simulink model "A13_Servoachse_Nyquist"  (R2017b)
settings: Solver=ode45  StartTime=0.0  StopTime=20  FixedStep=0.001  MaxStep=1E-3  RelTol=1e-3  EnableMultiTasking=on
values from neighbouring files (symbols this model uses):
  CF = 1e4    (= 10000)    [A13_Konstanten.m]    (also in A14_Konstanten.m; A17_Konstanten.m = 50000; A8_Konstanten.m = 10000000; A9_Konstanten.m)
  CM = 7.1e-7    (= 7.1e-07)    [A10_Konstanten.m]    (also in A13_Konstanten.m; A14_Konstanten.m; A16_Konstanten.m)
  CR = 0.2    [A13_Konstanten.m]    (also in A14_Konstanten.m; A17_Konstanten.m = 100; A9_Konstanten.m = 1; Z_Parametrisierung_Skript.m = [0.5,1,5])
  FReib = 0.5    [A13_Konstanten.m]    (also in A14_Konstanten.m)
  JM = JR + JG    (= 1.38e-06)    [A13_Konstanten.m]    (also in A14_Konstanten.m)
  JR = 1.32e-6    (= 1.32e-06)    [A10_Konstanten.m]    (also in A13_Konstanten.m; A14_Konstanten.m; A16_Konstanten.m; A9_Konstanten.m = 0.004)
  KM = 38.4e-3    (= 0.0384)    [A10_Konstanten.m]    (also in A13_Konstanten.m; A14_Konstanten.m; A16_Konstanten.m)
  KN = 1/(2*pi*KM)    (= 4.14465997635)    [A10_Konstanten.m]    (also in A13_Konstanten.m; A14_Konstanten.m; A16_Konstanten.m)
  LA = 4.64e-4    (= 0.000464)    [A10_Konstanten.m]    (also in A13_Konstanten.m; A14_Konstanten.m; A16_Konstanten.m)
  m1 = 1    [A13_Konstanten.m]    (also in A14_Konstanten.m; A17_Konstanten.m = 4; A8_Konstanten.m = 20)
  R = 0.02    [A10_Konstanten.m]    (also in A13_Konstanten.m = 0.04; A14_Konstanten.m = 0.04; A16_Konstanten.m)
  RA = 4.99    [A10_Konstanten.m]    (also in A13_Konstanten.m; A14_Konstanten.m; A16_Konstanten.m)
  Ue = 4    [A13_Konstanten.m]    (also in A14_Konstanten.m)
  UN = 24    [A13_Konstanten.m]    (also in A14_Konstanten.m)
  WGrad = 0.85    [A13_Konstanten.m]    (also in A14_Konstanten.m)
undefined symbols (not defined in the file or in its folder): sigbuilder_block
libraries: simulink x1
settings Model: Creator=jbaur  LastModifiedBy=lukasschwoerer
settings DataIOCC: ExternalInput=X1  SaveFormat=StructureWithTime  InspectSignalLogs=on  SignalLoggingName=sigsOut
settings OptimizationCC: DefaultParameterBehavior=Inlined  InlineInvariantSignals=on  BufferReuse=off  ExpressionDepthLimit=2147483647  InitFltsAndDblsToZero=on  LifeSpan=inf
settings DebuggingCC: SaveWithParameterizedLinksMsg=none  SignalResolutionControl=TryResolveAllWithWarning  MultiTaskDSMMsg=warning  MultiTaskCondExecSysMsg=none  StateNameClashWarn=warning  InitInArrayFormatMsg=none  SFUnexpectedBacktrackingDiag=warning  SFNoUnconditionalDefaultTransitionDiag=warning  SFExecutionAtInitializationDiag=none
settings HardwareCC: ProdBitPerPointer=32  ProdBitPerSizeT=32  ProdBitPerPtrDiffT=32  ProdLargestAtomicFloat=None  ProdIntDivRoundTo=Undefined  ProdEndianess=Unspecified  ProdWordSize=32  ProdHWDeviceType=32-bit Generic  TargetUnknown=on
settings ModelReferenceCC: PropagateSignalLabelsOutOfModel=off
settings CodeAppCC: StateflowObjectComments=on
settings GRTTargetCC: TargetFcnLib=ansi_tfl_tmw.mat  TargetLangStandard=C89/C90 (ANSI)  ModelReferenceCompliant=off  GeneratePreprocessorConditionals=Disable all  CombineOutputUpdateFcns=off  MatFileLogging=off  GRTInterface=on
settings ConfigComp: CovMetricSettings=dw  CovHtmlReporting=on  CovSaveCumulativeToWorkspaceVar=on  CovSaveSingleToWorkspaceVar=on  CovExternalEMLEnable=off  CovSFcnEnable=off

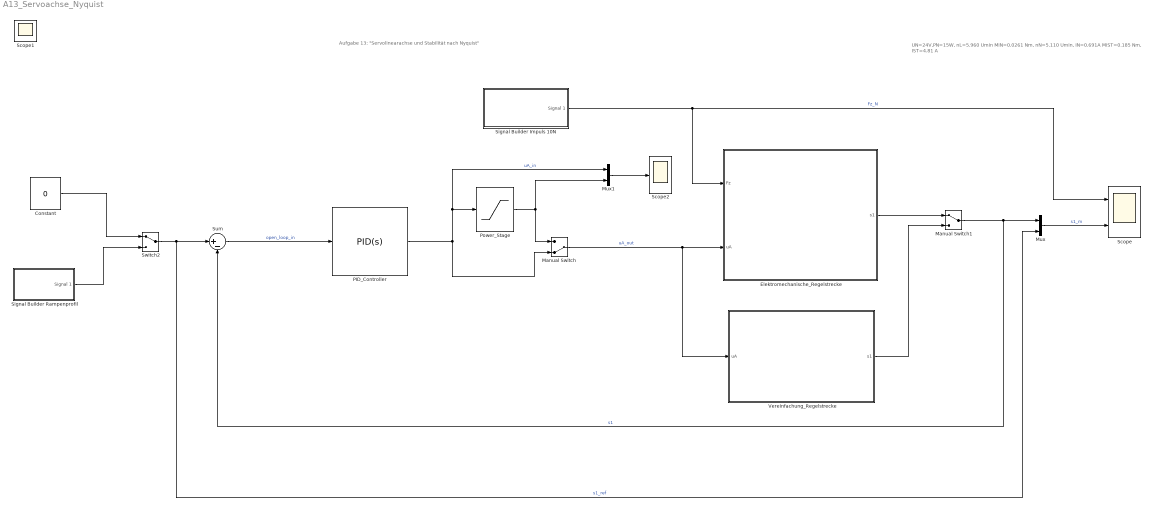
== system A13_Servoachse_Nyquist ==
  note: Aufgabe 13: "Servolinearachse und Stabilität nach Nyquist"
  note: UN=24V,PN=15W, nL=5.960 Umin
      | MiN=0.0261 Nm, nN=5.110 Umin, IN=0.691A
      | MiST=0.185 Nm, IST=4.81 A
  Constant : Constant  Value=0
  Elektromechanische_Regelstrecke : Subsystem
  Manual Switch : ManualSwitch  CurrentSetting=0
  Manual Switch1 : ManualSwitch
  Mux : Mux  Inputs=2
  Mux1 : Mux  Inputs=2
  PID_Controller : simulink/Continuous/PID Controller  Controller=PID  TimeDomain=Continuous-time  SampleTime=-1  IntegratorMethod=Forward Euler  FilterMethod=Forward Euler  Form=Ideal  UseFilter=on  ControllerParametersSource=internal  P=2480.03319241958  I=4.7969020161188  D=0.0477426789872327  N=295.112462731563  InitialConditionSource=internal  InitialConditionForIntegrator=0  InitialConditionForFilter=0  ExternalReset=none  LimitOutput=off  UpperSaturationLimit=UN  LowerSaturationLimit=-UN  LinearizeAsGain=off  AntiWindupMode=none  Kb=1  TrackingMode=off  Kt=1  PParamMin=[]  PParamMax=[]  IParamMin=[]  IParamMax=[]  DParamMin=[]  DParamMax=[]  NParamMin=[]  NParamMax=[]  KbParamMin=[]  KbParamMax=[]  KtParamMin=[]  KtParamMax=[]  POutMin=[]  POutMax=[]  IOutMin=[]  IOutMax=[]  DOutMin=[]  DOutMax=[]  NOutMin=[]  NOutMax=[]  KbOutMin=[]  KbOutMax=[]  KtOutMin=[]  KtOutMax=[]  IntegratorOutMin=[]  IntegratorOutMax=[]  FilterOutMin=[]  FilterOutMax=[]  SumOutMin=[]  SumOutMax=[]  SumI1OutMin=[]  SumI1OutMax=[]  SumI2OutMin=[]  SumI2OutMax=[]  SumI3OutMin=[]  SumI3OutMax=[]  SumDOutMin=[]  SumDOutMax=[]  SaturationOutMin=[]  SaturationOutMax=[]  IntegratorContinuousStateAttributes=''  IntegratorStateMustResolveToSignalObject=off  IntegratorRTWStateStorageClass=Auto  FilterContinuousStateAttributes=''  FilterStateMustResolveToSignalObject=off  FilterRTWStateStorageClass=Auto  DifferentiatorICPrevScaledInput=0  DifferentiatorOutMin=[]  DifferentiatorOutMax=[]  InitialConditionSetting=State (most efficient)  FilterDiffOutCoefMin=[]  FilterDiffOutCoefMax=[]  SumDenOutMin=[]  SumDenOutMax=[]  SumNumOutMin=[]  SumNumOutMax=[]  ReciprocalOutMin=[]  ReciprocalOutMax=[]  DivideOutMin=[]  DivideOutMax=[]  TunerSelectOption=Transfer Function Based (PID Tuner App)
  Power_Stage : Saturate  UpperLimit=UN  LowerLimit=-UN
  Scope : Scope  NumInputPorts=2
  Scope2 : Scope
  Signal Builder Impuls 10N : Subsystem  Tag=STV Subsys  LoadFcn=sigbuilder_block('load');  StartFcn=sigbuilder_block('start');  StopFcn=sigbuilder_block('stop');  ClipboardFcn=sigbuilder_block('clipboard');  mask(Sigbuilder block){tuvar=[0:10]}
      mask help: Simulink:masks:SigbuilderBlock_MD
      mask init:
      | if ~strcmp(get_param(bdroot(gcbh),'SimulationStatus'),'stopped') tuvar = sigbuilder_block('maskInit'); end
      settings: CopyFcn=sigbuilder_block('copy');  DeleteFcn=sigbuilder_block('delete');  ModelCloseFcn=sigbuilder_block('modelClose');  PreSaveFcn=sigbuilder_block('preSave');  PauseFcn=sigbuilder_block('pause');  ContinueFcn=sigbuilder_block('continue');  NameChangeFcn=sigbuilder_block('namechange');  OpenFcn=sigbuilder_block('open',[437 199 551 400 ]);  CloseFcn=sigbuilder_block('close');
      mask Display: plot(0, 0, 100, 100,[2, 2, 32, 32, 2], [68, 8, 8, 68, 68],[32, 2], [38, 38], [32, 19, 2],[53, 60, 44], [32, 17, 17, 2],[16, 16, 31, 31]);txt = getActiveGroup(gcbh);text(2, 100, txt,'verticalAlignment', 'top');
  Signal Builder Rampenprofil : Subsystem  Tag=STV Subsys  LoadFcn=sigbuilder_block('load');  StartFcn=sigbuilder_block('start');  StopFcn=sigbuilder_block('stop');  ClipboardFcn=sigbuilder_block('clipboard');  mask(Sigbuilder block){tuvar=[0:10]}
      mask help: Create and generate interchangeable groups of signals whose waveforms are piecewise linear.
      mask init:
      | if ~strcmp(get_param(bdroot(gcbh),'SimulationStatus'),'stopped') tuvar = sigbuilder_block('maskInit'); end
      settings: CopyFcn=sigbuilder_block('copy');  DeleteFcn=sigbuilder_block('delete');  ModelCloseFcn=sigbuilder_block('modelClose');  PreSaveFcn=sigbuilder_block('preSave');  PauseFcn=sigbuilder_block('pause')  ContinueFcn=sigbuilder_block('continue')  NameChangeFcn=sigbuilder_block('namechange');  OpenFcn=sigbuilder_block('open',[441.75 165.75 550.5 399.75 ]);  CloseFcn=sigbuilder_block('close');
      mask Display: plot(0, 0, 100, 100,[2, 2, 32, 32, 2], [68, 8, 8, 68, 68],[32, 2], [38, 38], [32, 19, 2],[53, 60, 44], [32, 17, 17, 2],[16, 16, 31, 31]);txt = getActiveGroup(gcbh);text(2, 100, txt,'verticalAlignment', 'top');
  Sum : Sum  Inputs=|+-  SaturateOnIntegerOverflow=on
  Switch2 : ManualSwitch
  Vereinfachung_Regelstrecke : Subsystem
  Scope1 : Scope
  wires:
  Sum/1 -> PID_Controller/1  "open_loop_in"
  Signal Builder Impuls 10N/1(Signal 1) -> Elektromechanische_Regelstrecke/1(Fz), Scope/1  "Fz_N"
  Switch2/1 -> Sum/1, Mux/2  "s1_ref"
  Constant/1 -> Switch2/1
  Signal Builder Rampenprofil/1(Signal 1) -> Switch2/2
  Mux/1 -> Scope/2  "s1_m"
  Power_Stage/1 -> Manual Switch/1, Mux1/2
  Manual Switch/1 -> Vereinfachung_Regelstrecke/1(uA), Elektromechanische_Regelstrecke/2(uA)  "uA_out"
  PID_Controller/1 -> Manual Switch/2, Mux1/1, Power_Stage/1  "uA_in"
  Mux1/1 -> Scope2/1
  Manual Switch1/1 -> Sum/2, Mux/1  "s1"
  Elektromechanische_Regelstrecke/1(s1) -> Manual Switch1/1
  Vereinfachung_Regelstrecke/1(s1) -> Manual Switch1/2

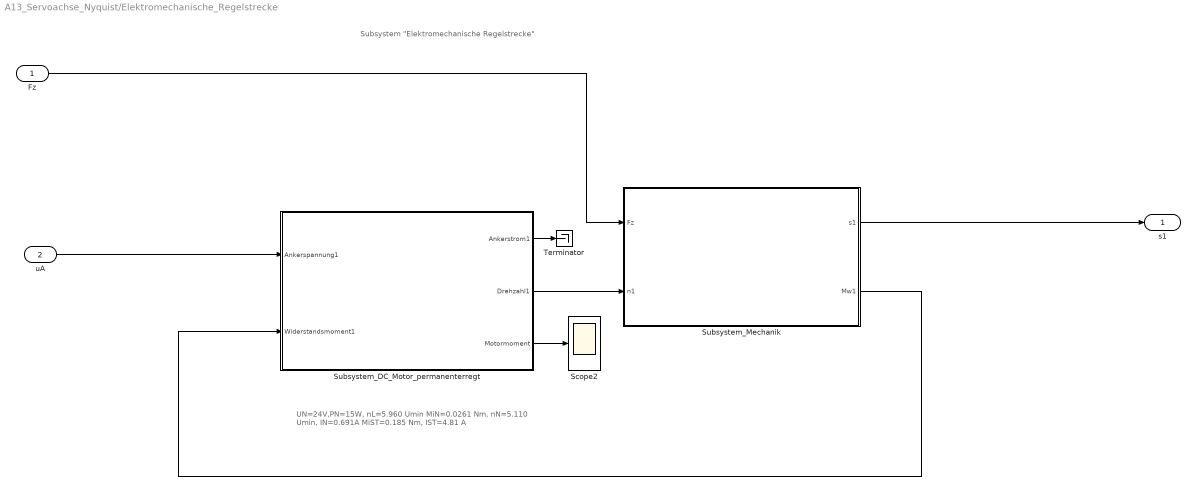
== system A13_Servoachse_Nyquist/Elektromechanische_Regelstrecke ==
  note: Subsystem "Elektromechanische Regelstrecke"
  note: UN=24V,PN=15W, nL=5.960 Umin
      | MiN=0.0261 Nm, nN=5.110 Umin, IN=0.691A
      | MiST=0.185 Nm, IST=4.81 A
  Fz : Inport
  uA : Inport  Port=2
  Scope2 : Scope
  Subsystem_DC_Motor_permanenterregt : Subsystem
  Subsystem_Mechanik : Subsystem
  Terminator : Terminator
  s1 : Outport
  wires:
  Fz/1 -> Subsystem_Mechanik/1(Fz)
  Subsystem_DC_Motor_permanenterregt/2(Drehzahl1) -> Subsystem_Mechanik/2(n1)
  Subsystem_Mechanik/2(Mw1) -> Subsystem_DC_Motor_permanenterregt/2(Widerstandsmoment1)
  Subsystem_Mechanik/1(s1) -> s1/1
  uA/1 -> Subsystem_DC_Motor_permanenterregt/1(Ankerspannung1)
  Subsystem_DC_Motor_permanenterregt/1(Ankerstrom1) -> Terminator/1
  Subsystem_DC_Motor_permanenterregt/3(Motormoment) -> Scope2/1

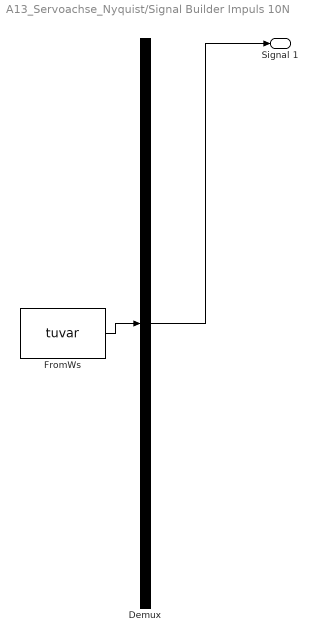
== system A13_Servoachse_Nyquist/Signal Builder Impuls 10N ==
  Demux : Demux  Tag=STV Demux  Outputs=1
  FromWs : FromWorkspace  Tag=STV FromWs  VariableName=tuvar  SampleTime=0
      SigBuilderData=|
      | common.afterFinalStr = 'Extrapolate'
      | common.sampleTime = 0
      | dataSet.timeRange = [0 20]
      | dataSet.name = 'Group 1'
      | sbobj.Groups.Name = 'Group 1'
      | sbobj.Groups.Signals.Name = 'Signal 1'
      | sbobj.Groups.Signals.XData = [0 10 10 11 11 20]
      | sbobj.Groups.Signals.YData = [0 0 10 10 0 0]
      | sbobj.Groups.TimeRange = [0 20]
  Signal 1 : Outport  Tag=STV Outport
  wires:
  Demux/1 -> Signal 1/1
  FromWs/1 -> Demux/1

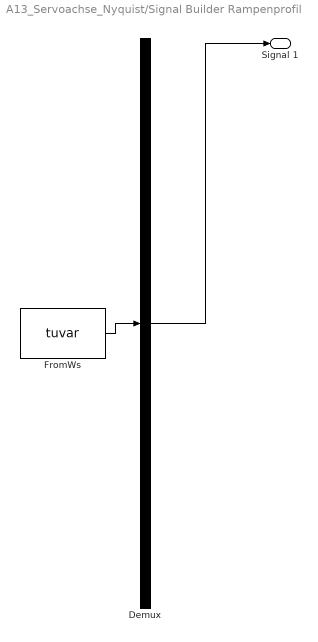
== system A13_Servoachse_Nyquist/Signal Builder Rampenprofil ==
  Demux : Demux  Tag=STV Demux  Outputs=1
  FromWs : FromWorkspace  Tag=STV FromWs  VariableName=tuvar  SampleTime=0
      SigBuilderData=|
      | common.afterFinalStr = 'Extrapolate'
      | common.sampleTime = 0
      | dataSet.timeRange = [0 10]
      | dataSet.name = 'Group 1'
      | sbobj.Groups.Name = 'Group 1'
      | sbobj.Groups.Signals.Name = 'Signal 1'
      | sbobj.Groups.Signals.XData = [0 2 3 5 6 10]
      | sbobj.Groups.Signals.YData = [0 0 0.5 0.5 0 0]
  Signal 1 : Outport  Tag=STV Outport
  wires:
  Demux/1 -> Signal 1/1
  FromWs/1 -> Demux/1

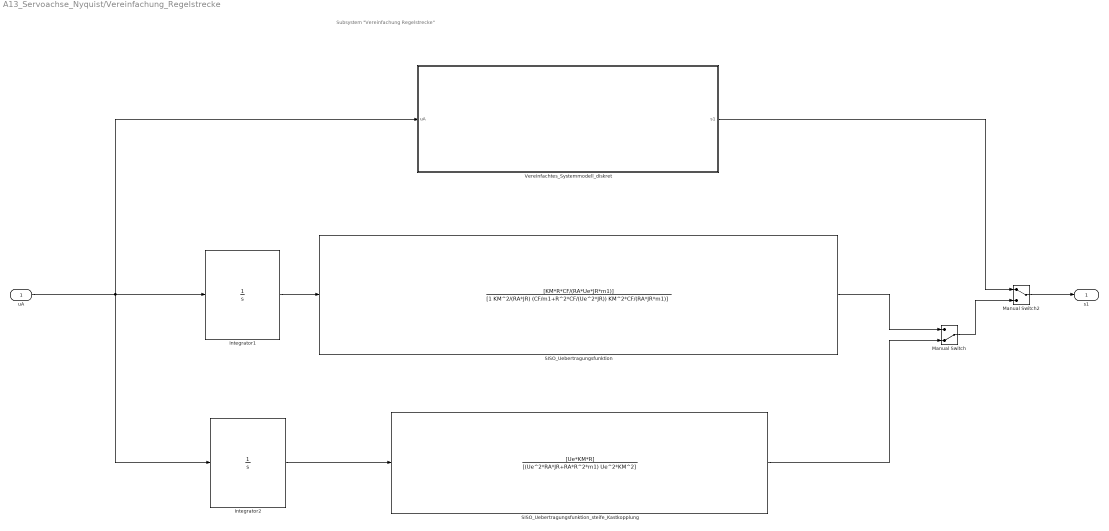
== system A13_Servoachse_Nyquist/Vereinfachung_Regelstrecke ==
  note: Subsystem "Vereinfachung Regelstrecke"
  uA : Inport
  Integrator1 : Integrator
  Integrator2 : Integrator
  Manual Switch : ManualSwitch  CurrentSetting=0
  Manual Switch2 : ManualSwitch
  SISO_Uebertragungsfunktion : TransferFcn  Numerator=[KM*R*CF/(RA*Ue*JR*m1)]  Denominator=[1 KM^2/(RA*JR) (CF/m1+R^2*CF/(Ue^2*JR)) KM^2*CF/(RA*JR*m1)]
  SISO_Uebertragungsfunktion_steife_Kastkopplung : TransferFcn  Numerator=[Ue*KM*R]  Denominator=[(Ue^2*RA*JR+RA*R^2*m1) Ue^2*KM^2]
  Vereinfachtes_Systemmodell_diskret : Subsystem
  s1 : Outport
  wires:
  Manual Switch2/1 -> s1/1
  Vereinfachtes_Systemmodell_diskret/1(s1) -> Manual Switch2/1
  Integrator2/1 -> SISO_Uebertragungsfunktion_steife_Kastkopplung/1
  uA/1 -> Vereinfachtes_Systemmodell_diskret/1(uA), Integrator1/1, Integrator2/1
  Integrator1/1 -> SISO_Uebertragungsfunktion/1
  Manual Switch/1 -> Manual Switch2/2
  SISO_Uebertragungsfunktion/1 -> Manual Switch/1
  SISO_Uebertragungsfunktion_steife_Kastkopplung/1 -> Manual Switch/2

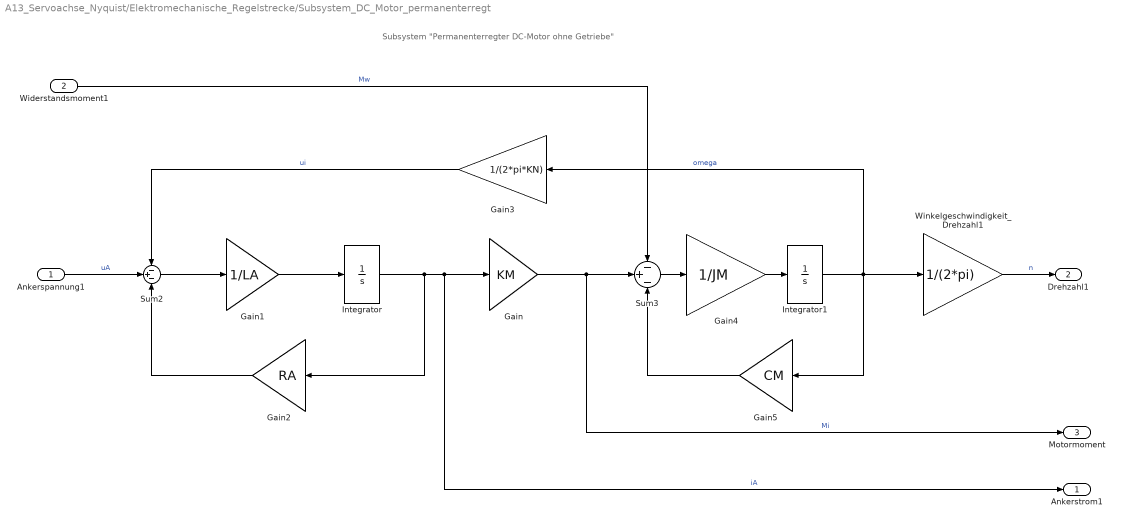
== system A13_Servoachse_Nyquist/Elektromechanische_Regelstrecke/Subsystem_DC_Motor_permanenterregt ==
  note: Subsystem "Permanenterregter DC-Motor ohne Getriebe"
  Ankerspannung1 : Inport
  Widerstandsmoment1 : Inport  Port=2
  Gain : Gain  Gain=KM
  Gain1 : Gain  Gain=1/LA
  Gain2 : Gain  Gain=RA
  Gain3 : Gain  Gain=1/(2*pi*KN)
  Gain4 : Gain  Gain=1/JM
  Gain5 : Gain  Gain=CM
  Integrator : Integrator
  Integrator1 : Integrator
  Sum2 : Sum  Inputs=-+-
  Sum3 : Sum  Inputs=-+-
  Winkelgeschwindigkeit_Drehzahl1 : Gain  Gain=1/(2*pi)
  Ankerstrom1 : Outport
  Drehzahl1 : Outport  Port=2
  Motormoment : Outport  Port=3
  wires:
  Ankerspannung1/1 -> Sum2/2  "uA"
  Gain3/1 -> Sum2/1  "ui"
  Gain/1 -> Sum3/2, Motormoment/1  "Mi"
  Winkelgeschwindigkeit_Drehzahl1/1 -> Drehzahl1/1  "n"
  Sum2/1 -> Gain1/1
  Gain1/1 -> Integrator/1
  Integrator/1 -> Gain2/1, Ankerstrom1/1, Gain/1  "iA"
  Sum3/1 -> Gain4/1
  Gain4/1 -> Integrator1/1
  Integrator1/1 -> Gain3/1, Winkelgeschwindigkeit_Drehzahl1/1, Gain5/1  "omega"
  Gain5/1 -> Sum3/3
  Gain2/1 -> Sum2/3
  Widerstandsmoment1/1 -> Sum3/1  "Mw"

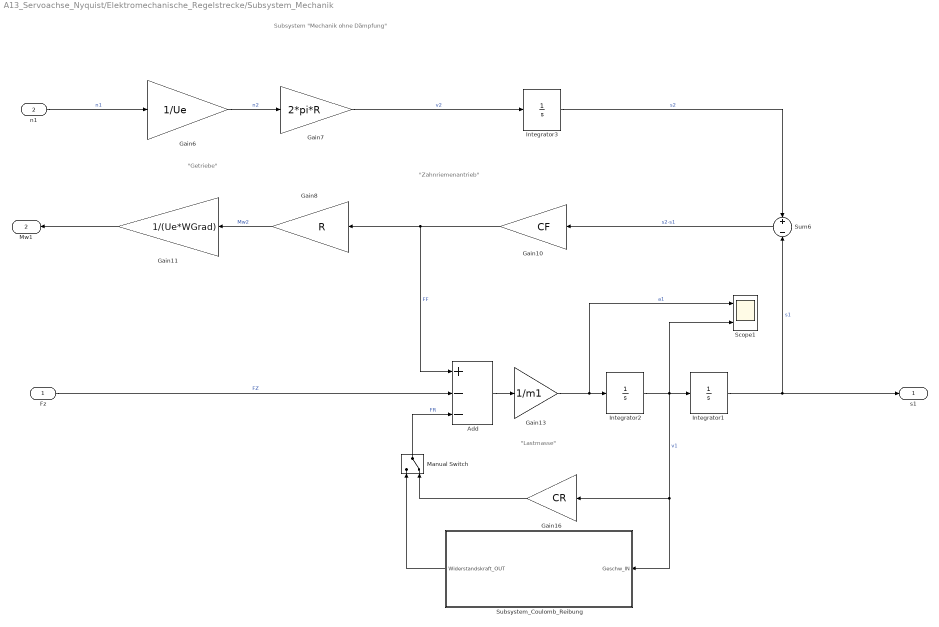
== system A13_Servoachse_Nyquist/Elektromechanische_Regelstrecke/Subsystem_Mechanik ==
  note: Subsystem "Mechanik ohne Dämpfung"
  note: "Lastmasse"
  note: "Zahnriemenantrieb"
  note: "Getriebe"
  Fz : Inport
  n1 : Inport  Port=2
  Add : Sum  Inputs=+--
  Gain10 : Gain  Gain=CF
  Gain11 : Gain  Gain=1/(Ue*WGrad)
  Gain13 : Gain  Gain=1/m1
  Gain16 : Gain  Gain=CR
  Gain6 : Gain  Gain=1/Ue
  Gain7 : Gain  Gain=2*pi*R
  Gain8 : Gain  Gain=R
  Integrator1 : Integrator
  Integrator2 : Integrator
  Integrator3 : Integrator
  Manual Switch : ManualSwitch  CurrentSetting=0
  Scope1 : Scope  NumInputPorts=2
  Subsystem_Coulomb_Reibung : Subsystem
  Sum6 : Sum  Inputs=+|-
  s1 : Outport
  Mw1 : Outport  Port=2
  wires:
  Integrator2/1 -> Scope1/2, Integrator1/1, Subsystem_Coulomb_Reibung/1(Geschw_IN), Gain16/1  "v1"
  Integrator1/1 -> s1/1, Sum6/2  "s1"
  Add/1 -> Gain13/1
  Gain13/1 -> Scope1/1, Integrator2/1  "a1"
  Gain7/1 -> Integrator3/1  "v2"
  Gain8/1 -> Gain11/1  "Mw2"
  Sum6/1 -> Gain10/1  "s2-s1"
  Integrator3/1 -> Sum6/1  "s2"
  Gain10/1 -> Gain8/1, Add/1  "FF"
  n1/1 -> Gain6/1  "n1"
  Gain6/1 -> Gain7/1  "n2"
  Fz/1 -> Add/2  "FZ"
  Gain11/1 -> Mw1/1
  Manual Switch/1 -> Add/3  "FR"
  Gain16/1 -> Manual Switch/2
  Subsystem_Coulomb_Reibung/1(Widerstandskraft_OUT) -> Manual Switch/1

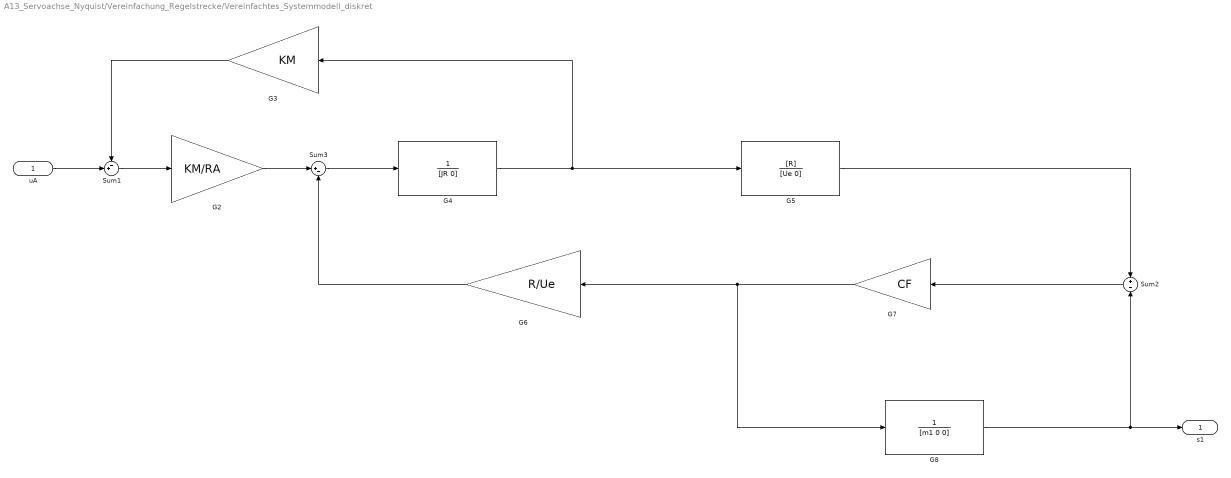
== system A13_Servoachse_Nyquist/Vereinfachung_Regelstrecke/Vereinfachtes_Systemmodell_diskret ==
  uA : Inport
  G2 : Gain  Gain=KM/RA
  G3 : Gain  Gain=KM
  G4 : TransferFcn  Denominator=[JR 0]
  G5 : TransferFcn  Numerator=[R]  Denominator=[Ue 0]
  G6 : Gain  Gain=R/Ue
  G7 : Gain  Gain=CF
  G8 : TransferFcn  Denominator=[m1 0 0]
  Sum1 : Sum  Inputs=-+|
  Sum2 : Sum  Inputs=+|-
  Sum3 : Sum  Inputs=|+-
  s1 : Outport
  wires:
  G2/1 -> Sum3/1
  G7/1 -> G8/1, G6/1
  Sum2/1 -> G7/1
  Sum1/1 -> G2/1
  G5/1 -> Sum2/1
  G4/1 -> G5/1, G3/1
  Sum3/1 -> G4/1
  uA/1 -> Sum1/2
  G3/1 -> Sum1/1
  G6/1 -> Sum3/2
  G8/1 -> s1/1, Sum2/2

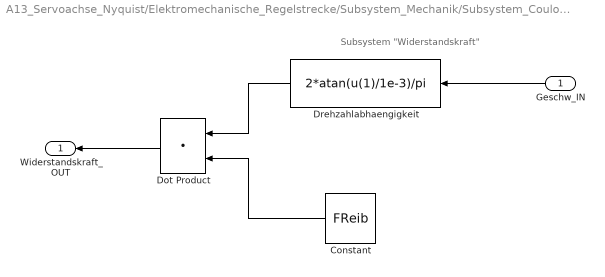
== system A13_Servoachse_Nyquist/Elektromechanische_Regelstrecke/Subsystem_Mechanik/Subsystem_Coulomb_Reibung ==
  note: Subsystem "Widerstandskraft"
  Geschw_IN : Inport
  Constant : Constant  Value=FReib
  Dot Product : DotProduct  InputSameDT=on  OutDataTypeStr=Inherit: Inherit via internal rule
  Drehzahlabhaengigkeit : Fcn  Expr=2*atan(u(1)/1e-3)/pi
  Widerstandskraft_OUT : Outport
  wires:
  Constant/1 -> Dot Product/2
  Drehzahlabhaengigkeit/1 -> Dot Product/1
  Geschw_IN/1 -> Drehzahlabhaengigkeit/1
  Dot Product/1 -> Widerstandskraft_OUT/1
